simulink model "model3"  (R2022a)
settings: Solver=FixedStepAuto  StartTime=0.0  StopTime=25  FixedStep=0.001  RelTol=1e-3
undefined symbols (not defined in the file): A, B, C, D, g, K, L, l1, l2, M, m1, m2, phi1_0, phi2_0, v_0, w1_0, w2_0, x0, x_0
settings Model: Creator=Дети  LastModifiedBy=Rynsi
settings ModelReferenceCC: EnableRefExpFcnMdlSchedulingChecks=off
settings RTWCC: Description=Generic Real-Time Target

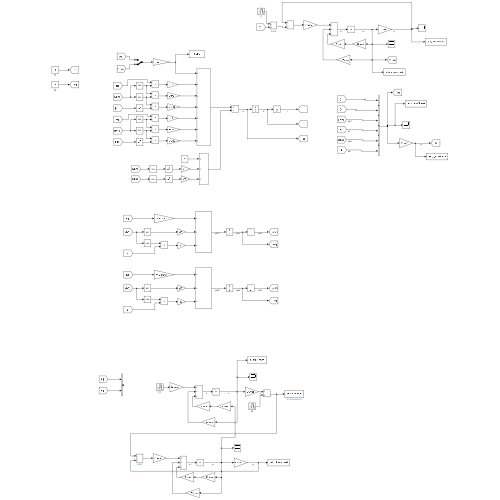
[thumbnail: Simulink's stored preview of the top-level diagram]
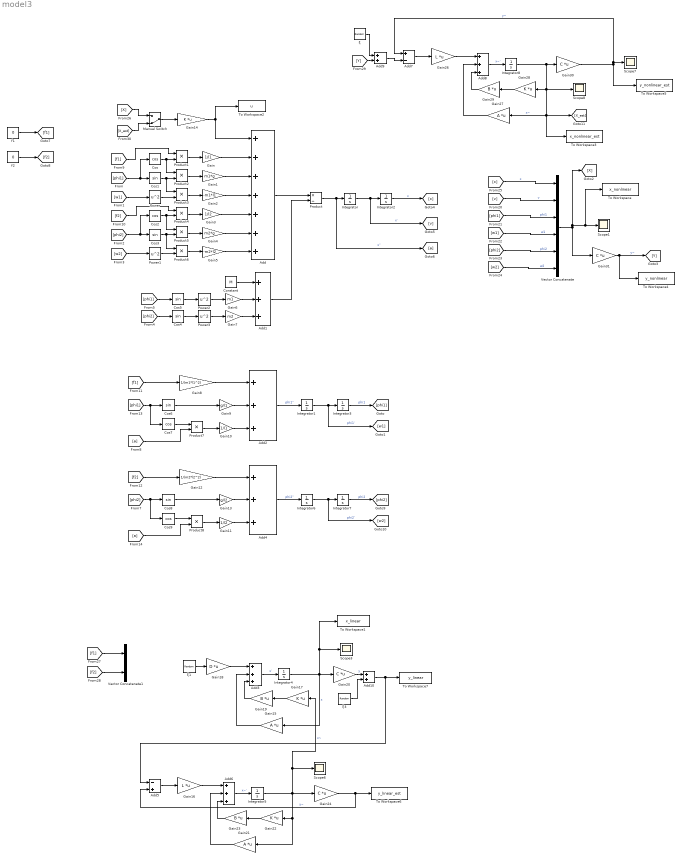
== system model3 ==
  Add : Sum  Inputs=+++++++
  Add{1..4,6,8} (6 alike) : Sum  Inputs=+++
  Add10 : Sum
  Add5 : Sum  Inputs=-+
  Add7 : Sum  Inputs=+-
  Add9 : Sum
  Constant : Constant  Value=M
  Cos{,2,7,9} (4 alike) : Trigonometry  Operator=cos
  Cos{1,3..6,8} (6 alike) : Trigonometry
  Gain : Gain  Gain=1/l1
  Gain1 : Gain  Gain=m1*g
  Gain10 : Gain  Gain=1/l1
  Gain11 : Gain  Gain=1/l2
  Gain12 : Gain  Gain=1/(m2*l2^2)
  Gain13 : Gain  Gain=g/l2
  Gain{14,17,22,28} (4 alike) : Gain  Gain=K  Multiplication=Matrix(K*u) (u vector)
  Gain15 : Gain  Gain=A  Multiplication=Matrix(K*u) (u vector)
  Gain16 : Gain  Gain=L  Multiplication=Matrix(K*u) (u vector)
  Gain18 : Gain  Gain=D  Multiplication=Matrix(K*u) (u vector)
  Gain19 : Gain  Gain=B  Multiplication=Matrix(K*u) (u vector)
  Gain2 : Gain  Gain=-m1*l1
  Gain{20,24,30..31} (4 alike) : Gain  Gain=C  Multiplication=Matrix(K*u) (u vector)
  Gain21 : Gain  Gain=A  Multiplication=Matrix(K*u) (u vector)
  Gain23 : Gain  Gain=B  Multiplication=Matrix(K*u) (u vector)
  Gain26 : Gain  Gain=L  Multiplication=Matrix(K*u) (u vector)
  Gain27 : Gain  Gain=A  Multiplication=Matrix(K*u) (u vector)
  Gain29 : Gain  Gain=B  Multiplication=Matrix(K*u) (u vector)
  Gain3 : Gain  Gain=1/l2
  Gain4 : Gain  Gain=m2*g
  Gain5 : Gain  Gain=-m2*l2
  Gain6 : Gain  Gain=m1
  Gain7 : Gain  Gain=m2
  Gain8 : Gain  Gain=1/(m1*l1^2)
  Gain9 : Gain  Gain=g/l1
  Integrator : Integrator  InitialCondition=v_0
  Integrator1 : Integrator  InitialCondition=w1_0
  Integrator2 : Integrator  InitialCondition=x_0
  Integrator3 : Integrator  InitialCondition=phi1_0
  Integrator4 : Integrator  InitialCondition=x0
  Integrator5 : Integrator  InitialCondition=x0
  Integrator6 : Integrator  InitialCondition=w2_0
  Integrator7 : Integrator  InitialCondition=phi2_0
  Integrator8 : Integrator  InitialCondition=x0
  Manual Switch : ManualSwitch  CurrentSetting=0
  Power{,1..3} (4 alike) : Math  Operator=square
  Product : Product  Inputs=*/
  Product{1..8} (8 alike) : Product
  Scope{1,3,6..8} (5 alike) : Scope
  To Workspace : ToWorkspace  VariableName=x_nonlinear  SaveFormat=Timeseries  SampleTime=-1
  To Workspace1 : ToWorkspace  VariableName=x_linear  SaveFormat=Timeseries  SampleTime=-1
  To Workspace2 : ToWorkspace  VariableName=u  SaveFormat=Timeseries  SampleTime=-1
  To Workspace3 : ToWorkspace  VariableName=x_nonlinear_est  SaveFormat=Timeseries  SampleTime=-1
  To Workspace4 : ToWorkspace  VariableName=y_nonlinear  SaveFormat=Timeseries  SampleTime=-1
  To Workspace5 : ToWorkspace  VariableName=y_nonlinear_est  SaveFormat=Timeseries  SampleTime=-1
  To Workspace6 : ToWorkspace  VariableName=y_linear_est  SaveFormat=Timeseries  SampleTime=-1
  To Workspace7 : ToWorkspace  VariableName=y_linear  SaveFormat=Timeseries  SampleTime=-1
  Vector Concatenate : Concatenate  NumInputs=6
  Vector Concatenate1 : Concatenate
  f1 : Constant  Value=0
  f2 : Constant  Value=0
  ξ : RandomNumber  Variance=2  Seed=[1,2,3]  SampleTime=0.01
  ξ1 : RandomNumber  Variance=3  Seed=[1,2]  SampleTime=0.01
  ξ3 : RandomNumber  Variance=0.1  Seed=[1,2,3]  SampleTime=0.01
  wires:
  Product/1 -> [a], Integrator/1  "x''"
  Integrator/1 -> [v], Integrator2/1  "x'"
  Add/1 -> Product/1
  Add1/1 -> Product/2
  Add2/1 -> Integrator1/1  "phi1''"
  Integrator1/1 -> [w1], Integrator3/1  "phi1'"
  Integrator2/1 -> [x]  "x"
  Integrator3/1 -> [phi1]  "phi1"
  [phi1] -> Cos/1, Cos1/1
  Cos/1 -> Product1/2, Product2/1
  [f1] -> Product1/1
  Product1/1 -> Gain/1
  Gain/1 -> Add/2
  Cos1/1 -> Product3/1, Product2/2
  Product2/1 -> Gain1/1
  [w1] -> Power/1
  Power/1 -> Product3/2
  Product3/1 -> Gain2/1
  Product6/1 -> Gain5/1
  Power1/1 -> Product6/2
  [w2] -> Power1/1
  Product5/1 -> Gain4/1
  Cos3/1 -> Product5/2, Product6/1
  Product4/1 -> Gain3/1
  [f2] -> Product4/1
  Cos2/1 -> Product5/1, Product4/2
  [phi2] -> Cos2/1, Cos3/1
  Constant/1 -> Add1/1
  Power2/1 -> Gain6/1
  Power3/1 -> Gain7/1
  Gain6/1 -> Add1/2
  [phi2] -> Cos4/1
  Cos4/1 -> Power3/1
  [phi1] -> Cos5/1
  Cos5/1 -> Power2/1
  f1/1 -> [f1]
  f2/1 -> [f2]
  [f1] -> Gain8/1
  [phi1] -> Cos7/1, Cos6/1
  Gain8/1 -> Add2/1
  Cos6/1 -> Gain9/1
  Gain9/1 -> Add2/2
  [a] -> Product7/2
  Product7/1 -> Gain10/1
  Cos7/1 -> Product7/1
  Cos9/1 -> Product8/1
  Product8/1 -> Gain11/1
  [a] -> Product8/2
  Gain13/1 -> Add4/2
  Cos8/1 -> Gain13/1
  Gain12/1 -> Add4/1
  [phi2] -> Cos8/1, Cos9/1
  [f2] -> Gain12/1
  Integrator7/1 -> [phi2]  "phi2"
  Integrator6/1 -> Integrator7/1, [w2]  "phi2'"
  Add4/1 -> Integrator6/1  "phi2''"
  [v] -> Vector Concatenate/2  "v"
  [x] -> Vector Concatenate/1  "x"
  Vector Concatenate/1 -> [X], To Workspace/1, Scope1/1, Gain31/1
  Gain14/1 -> Add/1, To Workspace2/1
  Add3/1 -> Integrator4/1  "x'"
  Integrator4/1 -> To Workspace1/1, Scope3/1, Gain20/1, Gain15/1  "x"
  Gain17/1 -> Gain19/1
  Gain15/1 -> Add3/2
  [f1] -> Vector Concatenate1/1
  [f2] -> Vector Concatenate1/2
  Gain18/1 -> Add3/1
  Gain19/1 -> Add3/3
  Gain24/1 -> To Workspace6/1, Add5/2  "y~"
  Gain23/1 -> Add6/3
  Gain16/1 -> Add6/1
  Gain21/1 -> Add6/2
  Gain22/1 -> Gain23/1
  Integrator5/1 -> Gain21/1, Gain22/1, Gain24/1, Gain17/1, Scope6/1  "x~"
  Add6/1 -> Integrator5/1  "x~'"
  Add5/1 -> Gain16/1
  Add7/1 -> Gain26/1
  Add8/1 -> Integrator8/1  "x~'"
  Integrator8/1 -> Gain28/1, To Workspace3/1, [X_est], Gain27/1, Scope8/1, Gain30/1  "x~"
  Gain28/1 -> Gain29/1
  Gain27/1 -> Add8/2
  Gain26/1 -> Add8/1
  Gain29/1 -> Add8/3
  Gain31/1 -> To Workspace4/1, [Y]  "y~"
  Manual Switch/1 -> Gain14/1
  [X] -> Manual Switch/1
  [X_est] -> Manual Switch/2
  Gain1/1 -> Add/3
  Gain2/1 -> Add/4
  Gain3/1 -> Add/5
  Gain4/1 -> Add/6
  Gain5/1 -> Add/7
  Gain7/1 -> Add1/3
  Gain10/1 -> Add2/3
  Gain11/1 -> Add4/3
  [phi1] -> Vector Concatenate/3  "phi1"
  [w1] -> Vector Concatenate/4  "w1"
  [phi2] -> Vector Concatenate/5  "phi2"
  [w2] -> Vector Concatenate/6  "w2"
  ξ1/1 -> Gain18/1
  Gain30/1 -> Scope7/1, Add7/1, To Workspace5/1  "y~"
  [Y] -> Add9/2
  ξ/1 -> Add9/1
  Add9/1 -> Add7/2
  Gain20/1 -> Add10/1  "y"
  Add10/1 -> To Workspace7/1, Add5/1
  ξ3/1 -> Add10/2
